simulink model "sampleModel1531"  (R2023a)
settings: Solver=VariableStepAuto  StartTime=0.0  StopTime=10.0  RelTol=1e-3
libraries: hdlsllib x4, simulink x2
settings Model: Creator=user1  LastModifiedBy=user1

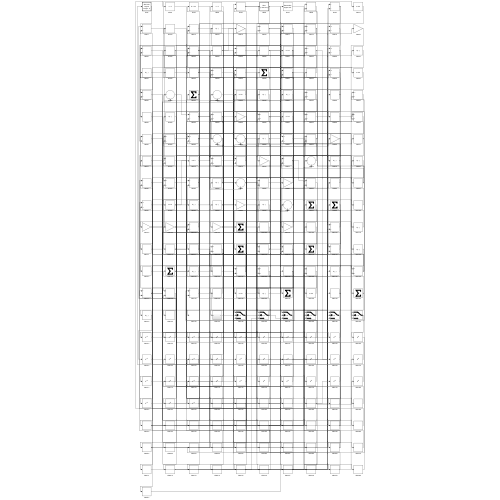
[thumbnail: Simulink's stored preview of the top-level diagram]
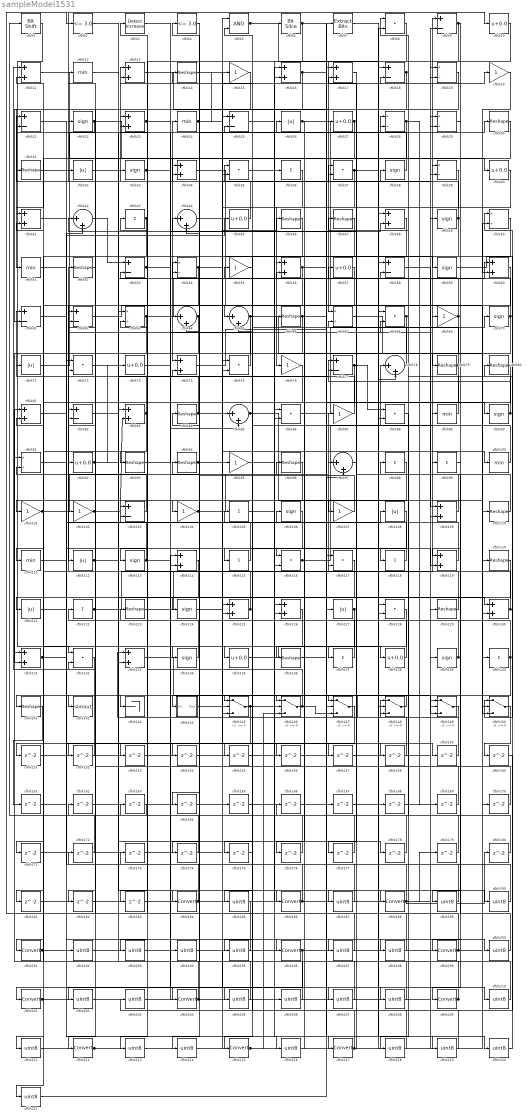
== system sampleModel1531 ==
  cfblk1 : hdlsllib/Logic and Bit Operations/Bit Shift  mode=Shift Left Logical  N=0
  cfblk{10,27,40,45,57,73,92,135,138} (9 alike) : Bias  Bias=0.0  SaturateOnIntegerOverflow=off
  cfblk{12,24,51,89,100,111} (6 alike) : MinMax
  cfblk{15,20,55,69,76,87,95,101..102,104,107} (11 alike) : Gain
  cfblk{9,18,21,25,53,58,61..62,77,82,103} (11 alike) : Sum  Inputs=+-
  cfblk{36,43,98..99,105,115,118,122,137,140} (10 alike) : Sum  Inputs=+
  cfblk{22,33,38,49,59,70,90,106,113,124,134,139} (12 alike) : Signum
  cfblk{26,32,71,108,112,121,127} (7 alike) : Abs  SaturateOnIntegerOverflow=off
  cfblk{11,13,16..17,23,34,41,48,56,60,74,81,83,109,114,119,125..126,130..131,133} (21 alike) : Sum
  cfblk{14,30..31,46..47,52,66,79..80,84,93..94,96,110,120,123,129,136,141} (19 alike) : Reshape
  cfblk{8,35,37,68,72,75,86,88,116..117,128,132} (12 alike) : DotProduct  OutDataTypeStr=Inherit: Inherit via internal rule
  cfblk142 : ToWorkspace  VariableName=simout  SaveFormat=Timeseries  SampleTime=-1
  cfblk143 : Terminator
  cfblk144 : Subsystem
      settings: LibrarySourceBlock=|
      | hdlsllib/Ports &
      | Subsystems/Subsystem
  cfblk{145..150} (6 alike) : Switch  SaturateOnIntegerOverflow=off  InputSameDT=off
  cfblk{151..183} (33 alike) : Delay  SampleTime=1
  cfblk{184,186,188,191,196,199,201,204,209,212,215,217} (12 alike) : DataTypeConversion  SaturateOnIntegerOverflow=off  RndMeth=Floor
  cfblk{185,187,189..190,192..195,197..198,200,202..203,205..208,210..211,213..214,216,218..221} (26 alike) : DataTypeConversion  OutDataTypeStr=uint8  SaturateOnIntegerOverflow=off  RndMeth=Floor
  cfblk{19,28..29,39,50,54,63,67,91} (9 alike) : Product  Inputs=*/  RndMeth=Zero  SaturateOnIntegerOverflow=on
  cfblk2 : hdlsllib/Logic and Bit Operations/Compare To Constant  relop=<=  const=3.0  OutDataTypeStr=boolean
  cfblk3 : simulink/Logic and Bit Operations/Detect Increase  vinit=0.0  OutDataTypeStr=boolean
      settings: LibrarySourceBlock=|
      | hdlsllib/Logic and Bit
      | Operations/Detect
      | Increase
  cfblk4 : hdlsllib/Logic and Bit Operations/Compare To Constant  relop=<=  const=3.0  OutDataTypeStr=boolean
  cfblk{42,44,64..65,78,85,97} (7 alike) : Sum  Inputs=|++
  cfblk5 : Logic  AllPortsSameDT=off  OutDataTypeStr=boolean
  cfblk6 : hdlsllib/Logic and Bit Operations/Bit Slice  lidx=7  ridx=0
  cfblk7 : simulink/Logic and Bit Operations/Extract Bits  bitsToExtract=Upper half  numBits=8  bitIdxRange=[0 7]  outScalingMode=Preserve fixed-point scaling
      settings: LibrarySourceBlock=|
      | hdlsllib/Logic and Bit
      | Operations/Extract Bits
  wires:
  cfblk81/1 -> cfblk204/1
  cfblk8/1 -> cfblk113/1
  cfblk86/1 -> cfblk70/1
  cfblk122/1 -> cfblk87/1, cfblk77/1
  cfblk22/1 -> cfblk40/1, cfblk21/2
  cfblk25/1 -> cfblk217/1
  cfblk120/1 -> cfblk143/1
  cfblk134/1 -> cfblk123/1
  cfblk10/1 -> cfblk67/1
  cfblk133/1 -> cfblk146/1
  cfblk1/1 -> cfblk132/1
  cfblk71/1 -> cfblk28/1
  cfblk27/1 -> cfblk74/1, cfblk145/3
  cfblk125/1 -> cfblk52/1, cfblk44/2
  cfblk62/1 -> cfblk65/1
  cfblk80/1 -> cfblk112/1
  cfblk116/1 -> cfblk78/1, cfblk66/1
  cfblk49/1 -> cfblk24/1, cfblk142/1
  cfblk42/1 -> cfblk53/1
  cfblk68/1 -> cfblk38/1, cfblk116/2
  cfblk59/1 -> cfblk150/1
  cfblk112/1 -> cfblk30/1, cfblk96/1
  cfblk104/1 -> cfblk89/1, cfblk158/1
  cfblk32/1 -> cfblk13/1
  cfblk31/1 -> cfblk10/1
  cfblk54/1 -> cfblk82/1, cfblk20/1
  cfblk110/1 -> cfblk54/1
  cfblk145/1 -> cfblk97/1, cfblk193/1
  cfblk53/1 -> cfblk26/1, cfblk197/1
  cfblk135/1 -> cfblk138/1
  cfblk82/1 -> cfblk60/1
  cfblk24/1 -> cfblk15/1, cfblk28/2
  cfblk26/1 -> cfblk110/1, cfblk116/1, cfblk118/1
  cfblk19/1 -> cfblk212/1
  cfblk123/1 -> cfblk9/1
  cfblk38/1 -> cfblk4/1
  cfblk128/1 -> cfblk191/1
  cfblk69/1 -> cfblk17/2, cfblk176/1, cfblk177/1
  cfblk111/1 -> cfblk115/1
  cfblk6/1 -> cfblk149/3, cfblk183/1
  cfblk13/1 -> cfblk95/1
  cfblk52/1 -> cfblk92/1
  cfblk50/1 -> cfblk107/1
  cfblk74/1 -> cfblk17/1
  cfblk37/1 -> cfblk136/1, cfblk145/2, cfblk190/1
  cfblk44/1 -> cfblk59/1
  cfblk40/1 -> cfblk137/1
  cfblk118/1 -> cfblk32/1
  cfblk138/1 -> cfblk122/1
  cfblk102/1 -> cfblk83/2, cfblk178/1
  cfblk89/1 -> cfblk47/1
  cfblk127/1 -> cfblk205/1, cfblk214/1
  cfblk9/1 -> cfblk119/1, cfblk86/2
  cfblk16/1 -> cfblk134/1, cfblk90/1, cfblk130/1
  cfblk136/1 -> cfblk18/2
  cfblk114/1 -> cfblk201/1
  cfblk70/1 -> cfblk8/1, cfblk213/1
  cfblk109/1 -> cfblk42/1
  cfblk36/1 -> cfblk76/1
  cfblk83/1 -> cfblk61/1, cfblk111/1
  cfblk77/1 -> cfblk145/1, cfblk88/1
  cfblk131/1 -> cfblk108/1, cfblk103/2
  cfblk101/1 -> cfblk16/1, cfblk45/1
  cfblk3/1 -> cfblk119/2
  cfblk119/1 -> cfblk98/1
  cfblk108/1 -> cfblk126/2
  cfblk149/1 -> cfblk148/1
  cfblk67/1 -> cfblk140/1
  cfblk39/1 -> cfblk56/1
  cfblk97/1 -> cfblk67/2
  cfblk20/1 -> cfblk60/2
  cfblk12/1 -> cfblk186/1
  cfblk87/1 -> cfblk43/1
  cfblk66/1 -> cfblk79/1, cfblk175/1
  cfblk132/1 -> cfblk11/1
  cfblk99/1 -> cfblk199/1
  cfblk58/1 -> cfblk109/1
  cfblk63/1 -> cfblk36/1, cfblk23/1, cfblk182/1
  cfblk11/1 -> cfblk75/2
  cfblk18/1 -> cfblk51/1, cfblk164/1
  cfblk34/1 -> cfblk150/2
  cfblk30/1 -> cfblk64/1
  cfblk139/1 -> cfblk84/1, cfblk189/1
  cfblk79/1 -> cfblk93/1, cfblk37/1, cfblk37/2, cfblk181/1
  cfblk84/1 -> cfblk74/2, cfblk149/2, cfblk100/1
  cfblk56/1 -> cfblk117/1, cfblk104/1, cfblk198/1
  cfblk113/1 -> cfblk22/1, cfblk208/1
  cfblk65/1 -> cfblk120/1, cfblk131/2
  cfblk93/1 -> cfblk69/1
  cfblk100/1 -> cfblk13/2
  cfblk106/1 -> cfblk215/1
  cfblk75/1 -> cfblk62/1
  cfblk43/1 -> cfblk101/1, cfblk23/2
  cfblk2/1 -> cfblk184/1
  cfblk126/1 -> cfblk135/1
  cfblk94/1 -> cfblk46/1, cfblk68/2
  cfblk14/1 -> cfblk27/1
  cfblk107/1 -> cfblk14/1
  cfblk45/1 -> cfblk21/1
  cfblk137/1 -> cfblk5/2
  cfblk46/1 -> cfblk64/2
  cfblk48/1 -> cfblk144/1(In1)
  cfblk117/1 -> cfblk121/1
  cfblk146/1 -> cfblk63/2, cfblk147/3
  cfblk115/1 -> cfblk34/1
  cfblk129/1 -> cfblk31/1
  cfblk140/1 -> cfblk44/1, cfblk141/1
  cfblk73/1 -> cfblk48/2
  cfblk29/1 -> cfblk209/1
  cfblk90/1 -> cfblk34/2, cfblk77/2
  cfblk28/1 -> cfblk41/1, cfblk169/1
  cfblk144/1(Out1) -> cfblk39/1
  cfblk103/1 -> cfblk41/2
  cfblk17/1 -> cfblk147/1
  cfblk130/1 -> cfblk103/1, cfblk71/1, cfblk50/1
  cfblk64/1 -> cfblk152/1, cfblk153/1
  cfblk148/1 -> cfblk133/1
  cfblk33/1 -> cfblk3/1, cfblk85/2
  cfblk15/1 -> cfblk61/2
  cfblk5/1 -> cfblk58/1, cfblk6/1
  cfblk35/1 -> cfblk147/2
  cfblk91/1 -> cfblk196/1
  cfblk72/1 -> cfblk188/1
  cfblk92/1 -> cfblk124/1, cfblk73/1
  cfblk78/1 -> cfblk35/1
  cfblk23/1 -> cfblk125/2, cfblk130/2
  cfblk85/1 -> cfblk150/3, cfblk187/1
  cfblk98/1 -> cfblk151/1
  cfblk151/1 -> cfblk16/2
  cfblk152/1 -> cfblk131/1
  cfblk153/1 -> cfblk8/2
  cfblk96/1 -> cfblk154/1
  cfblk154/1 -> cfblk5/1
  cfblk76/1 -> cfblk155/1
  cfblk155/1 -> cfblk146/2
  cfblk124/1 -> cfblk156/1
  cfblk156/1 -> cfblk9/2
  cfblk121/1 -> cfblk157/1
  cfblk157/1 -> cfblk117/2
  cfblk158/1 -> cfblk63/1
  cfblk61/1 -> cfblk159/1
  cfblk159/1 -> cfblk125/1
  cfblk150/1 -> cfblk160/1
  cfblk141/1 -> cfblk161/1
  cfblk161/1 -> cfblk42/2
  cfblk162/1 -> cfblk75/1
  cfblk163/1 -> cfblk1/1
  cfblk164/1 -> cfblk54/2
  cfblk165/1 -> cfblk39/2
  cfblk166/1 -> cfblk48/1
  cfblk167/1 -> cfblk149/1
  cfblk168/1 -> cfblk148/3
  cfblk169/1 -> cfblk148/2
  cfblk170/1 -> cfblk62/2
  cfblk57/1 -> cfblk171/1
  cfblk171/1 -> cfblk85/1
  cfblk172/1 -> cfblk11/2
  cfblk4/1 -> cfblk174/1
  cfblk174/1 -> cfblk132/2
  cfblk175/1 -> cfblk65/2
  cfblk176/1 -> cfblk53/2
  cfblk177/1 -> cfblk82/2
  cfblk178/1 -> cfblk56/2
  cfblk179/1 -> cfblk58/2
  cfblk180/1 -> cfblk86/1
  cfblk181/1 -> cfblk133/2
  cfblk182/1 -> cfblk109/2
  cfblk183/1 -> cfblk126/1
  cfblk184/1 -> cfblk33/1, cfblk127/1
  cfblk47/1 -> cfblk185/1
  cfblk185/1 -> cfblk2/1
  cfblk186/1 -> cfblk172/1, cfblk219/1
  cfblk187/1 -> cfblk12/1
  cfblk188/1 -> cfblk180/1, cfblk179/1, cfblk102/1
  cfblk189/1 -> cfblk72/1
  cfblk190/1 -> cfblk72/2
  cfblk191/1 -> cfblk168/1, cfblk167/1, cfblk97/2
  cfblk41/1 -> cfblk192/1
  cfblk192/1 -> cfblk128/1
  cfblk193/1 -> cfblk128/2
  cfblk173/1 -> cfblk194/1
  cfblk55/1 -> cfblk195/1
  cfblk195/1 -> cfblk173/1
  cfblk196/1 -> cfblk50/2, cfblk78/2, cfblk211/1
  cfblk197/1 -> cfblk91/1
  cfblk198/1 -> cfblk91/2
  cfblk199/1 -> cfblk163/1, cfblk162/1
  cfblk51/1 -> cfblk200/1
  cfblk200/1 -> cfblk99/1
  cfblk201/1 -> cfblk35/2, cfblk139/1
  cfblk60/1 -> cfblk202/1
  cfblk202/1 -> cfblk114/1
  cfblk160/1 -> cfblk203/1
  cfblk203/1 -> cfblk114/2
  cfblk204/1 -> cfblk129/1, cfblk83/1
  cfblk205/1 -> cfblk81/1
  cfblk95/1 -> cfblk206/1
  cfblk206/1 -> cfblk81/2
  cfblk105/1 -> cfblk207/1
  cfblk207/1 -> cfblk94/1
  cfblk208/1 -> cfblk105/1
  cfblk209/1 -> cfblk68/1, cfblk55/1
  cfblk194/1 -> cfblk210/1
  cfblk210/1 -> cfblk29/1
  cfblk211/1 -> cfblk29/2
  cfblk212/1 -> cfblk165/1, cfblk18/1
  cfblk213/1 -> cfblk19/1
  cfblk214/1 -> cfblk19/2
  cfblk215/1 -> cfblk88/2, cfblk146/3
  cfblk21/1 -> cfblk216/1
  cfblk216/1 -> cfblk106/1
  cfblk217/1 -> cfblk170/1, cfblk166/1, cfblk57/1, cfblk49/1
  cfblk88/1 -> cfblk218/1
  cfblk218/1 -> cfblk25/1
  cfblk219/1 -> cfblk25/2
  cfblk7/1 -> cfblk220/1
  cfblk220/1 -> cfblk80/1
  cfblk147/1 -> cfblk221/1
  cfblk221/1 -> cfblk7/1

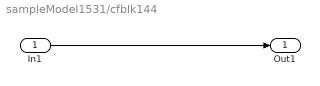
== system sampleModel1531/cfblk144 ==
  In1 : Inport
  Out1 : Outport
  wires:
  In1/1 -> Out1/1
